simulink model "T"  (R2022b)
settings: Solver=VariableStepAuto  StartTime=0.0  StopTime=10.0  RelTol=1e-3
settings Model: Creator=Milosh Yokich  LastModifiedBy=Milosh Yokich

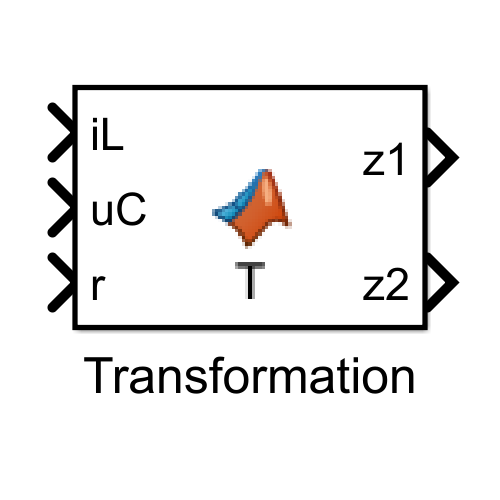
[thumbnail: Simulink's stored preview of the top-level diagram]
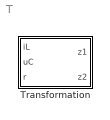
== system T ==
  Transformation : MATLAB Function  TreatAsAtomicUnit=on

== matlab function T/Transformation ==
  data: iL input; z1 output; uC input; r input; z2 output
function [z1, z2] = T(iL, uC, r)
E = 12; %V
R = 52; %Omh
L = 0.01591; %H
C = 0.000470; %F 

uCe = r;
ue = -(uCe)/(E-uCe);
iLe = -uCe/R/(1-ue);

gamma = L*1/2*iLe^2 + C*1/2*(uCe - E)^2;
gamma = -gamma;

% z1 = h(x)
z1 = L*1/2*iL^2 + C*1/2*uC^2 + gamma;
% z2 = Lf h(x)
z2 = E*(iL + uC/R) - uC/R*uC;
